simulink model "Galvo_sys_C__cont___Pcont_ccvc_FET_SUB_REF_v66"  (R2013a)
settings: Solver=ode23s  StartTime=0.0  StopTime=15e-3  FixedStep=FS  RelTol=1e-3
PreLoadFcn:
  | vname=@(x) inputname(1);
  | paramCtrl=evalin('base','paramCtrl;');
  | I_LIM=str2num(paramCtrl.I_LIM);
  | Kbc=str2num(paramCtrl.Kbc);
  | FS=evalin('base','FS;');
InitFcn:
  | %%%%%%  set scope time range
  | T_STOP=str2num(get_param(gcs,'StopTime'));
  | if numel(T_STOP) > 1
  |    T_STOP=T_STOP(2);
  | else
  |    T_STOP=T_STOP(1);
  | end
  | T_STOP=num2str(T_STOP);
  | 
  | %%%%%%  set scope time range in system @init_callback_fct
  | T_STOP=num2str(str2num(get_param(gcs,'StopTime')));
  | 
  | childs = allchild(0);
  | sol=strfind(upper(get(allchild(0),'Tag')),'VIEWER_PARAMETERS');
  | 
  | if iscell(sol)
  |    ind=find(~cellfun(@isempty, strfind(upper(get(allchild(0),'Tag')),'VIEWER_PARAMETERS')));
  | else
  |    ind=sol;
  | end
  | %ind=find(~cellfun(@isempty, {strfind(upper(get(allchild(0),'Tag')),'VIEWER_PARAMETERS'),[]}))
  | if ~isempty(ind)
  |    for k=1:length(childs(ind))
  |       set_param(getfield(get(childs(ind(k)),'UserData'),'block'),'TimeRange',T_STOP);
  |       get_param(getfield(get(childs(ind(k)),'UserData'),'block'),'TimeRange');
  | %    set_param(getfield(get(childs(ind),'UserData'),'block'),'TimeRange',T_STOP);
  | %    get_param(getfield(get(childs(ind),'UserData'),'block'),'TimeRange');
  |    end
  | else
  |     warning(sprintf('VIEWER_PARAMETERS object not found\nOpen the config dialog by hand for the first sim start'))
  | end
  | 
  | 
  | ADCres = str2num(get_param(gcs,'ADCres'));
  | Aref = str2num(get_param(gcs,'Aref'));
StartFcn:
  | I_LIM=str2num(paramCtrl.I_LIM);
  | Kbc=str2num(paramCtrl.Kbc);
  | %FS=evalin('base','FS;');
  | 
  | 
  | ADCres = str2num(get_param(gcs,'ADCres'));
  | Aref = str2num(get_param(gcs,'Aref'));
undefined symbols (not defined in the file or in its folder): ccG0, JR, KBM, KFR, KMT, KTB, Lc, Rc, Rsh
libraries: simulink x10, dspsigops x1
Description:
  | Eigentlich sollte in diesem Modell als current comp. ein ref. block mit zwei Varianten "alte 12V endstufe" und "neue 30V endstufe" eingesetzt werden. Sobald ein subsystem als referenced model eingesetzt wird, kommen die warnungen wegen algebr. schleifen obwohl sich die Blockdiagramme nicht unterscheiden.
  | --> anstatt "referenced variants" kommt halt wieder ein "subsystem variants" block als
  | cc rein...
settings Model: Aref=2.5  ADCres=12  BufferReuse=off  Creator=mainster  LastModifiedBy=mainster
settings SolverCC: AutoInsertRateTranBlk=on
settings DataIOCC: LimitDataPoints=off  SaveOutput=off  SaveTime=off
settings OptimizationCC: BlockReduction=off  InlineParams=on  OptimizeBlockIOStorage=off  BufferReuse=off  ExpressionFolding=off  LocalBlockOutputs=off
settings DebuggingCC: SolverPrmCheckMsg=none  InitInArrayFormatMsg=none
settings ModelReferenceCC: ModelReferenceNumInstancesAllowed=Single  ModelReferenceMinAlgLoopOccurrences=on

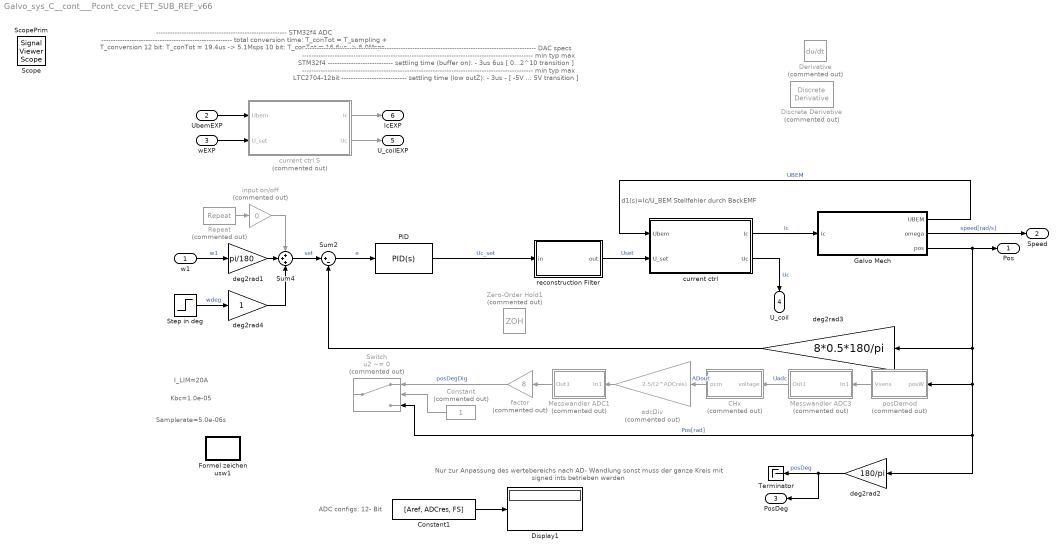
== system Galvo_sys_C__cont___Pcont_ccvc_FET_SUB_REF_v66 ==
  note: --------------------------------------------------------
      |  STM32f4 	ADC
      | --------------------------------------------------------
      | total conversion time:
      | T_conTot = T_sampling + T_conversion
      |
      | 12 bit: T_conTot = 19.4us -> 5.1Msps
      | 10 bit: T_conTot = 16.6us -> 6.0Msps
  note: Nur zur Anpassung des wertebereichs nach AD- Wandlung
      | sonst muss der ganze Kreis mit signed ints betrieben werden
  note: I_LIM=20A
  note: Kbc=1.0e-05
  note: Samplerate=5.0e-06s
  note: d1(s)=Ic/U_BEM
      | Stellfehler durch BackEMF
  note: ADC configs:
      | 12- Bit
  note: ---------------------------------------------------------------------------------------------------
      |  DAC specs
      | ---------------------------------------------------------------------------------------------------
      | 										min	typ		max
      | STM32f4							  ----------------------------
      | settling time (buffer on):	   -		3us	6us	[ 0...2^10 transition ]
      |
      | ---------------------------------------------------------------------------------------------------
      | 										min	typ		max
      | LTC2704-12bit 					  ----------------------------
      | settling time (low outZ):	   -		3us	-		[ -5V ... 5V transition ]
  w1 : Inport
  UbemEXP : Inport  Port=2
  wEXP : Inport  Port=3
  CHx : Subsystem  Commented=on  mask{bypass=off, N=eval(get_param(gcs,'ADCres'))}
      mask prompts: bypass "bypass adc"; N "Resolution"
      mask Callback bypass: %Simulink.Block.eval([gcb '/switch']);
      mask Callback N:
      | %va=strsplit(get_param(gcb, 'MaskVariables'), ';');
      | %ind=find(~cellfun(@isempty, strfind(va,'N')));
      | %sp=strsplit(va{ind},'=');
      | %@1
      | %set_param(gcs,'ADCres', @1)
      | %get_param(gcb, 'MaskVariables')
      mask Display:
      | %fprintf('ADC\nGain=%s\n=%i',...
      | %    get_param([gcb '/scale'], 'Gain'),...
      | %    eval( get_param([gcb '/scale'], 'Gain') ));
      | if bypass
      |     color('red')
      |     fprintf('bypass\nADC\n%i Bit', N)
      | else
      |     color('black')
      |     fprintf('ADC\n%i Bit', N)
      | end
  Constant : Constant  Commented=on
  Constant1 : Constant  Value=[Aref, ADCres, FS]
  Derivative : Derivative  Commented=on
  Discrete Derivative : simulink/Discrete/Discrete Derivative  Commented=on  gainval=1.0  ICPrevScaledInput=0.0  InputProcessing=Inherited  OutMin=[]  OutMax=[]  OutDataType=fixdt(1, 16)  OutScaling=2^-10  DoSatur=off
  Display1 : Display
  Formel zeichen usw1 : Subsystem
  Galvo Mech : Subsystem
  Messwandler ADC1 : Subsystem  Commented=on  mask{bias=-1.25, fact=1}
      mask prompts: bias "Enter offset"; fact "factor"
      mask TypeOptions bias: bias/Value
      mask TypeOptions fact: input div/Gain
      mask Display:
      | if bias < 0
      |     fprintf('y=%.4g*x%.4g',fact,bias)
      | else
      |     fprintf('y=%.4g*x+%.4g',fact,bias)
      | end
      | %port_label('input', 1, 'Vsens','texmode','off')
      | %port_label('output', 1, 'Vadc','texmode','off')
  Messwandler ADC3 : Subsystem  Commented=on  mask{bias=1.25, fact=1/4}
      mask prompts: bias "Enter offset"; fact "factor"
      mask TypeOptions bias: bias/Value
      mask TypeOptions fact: input div/Gain
      mask Display:
      | if bias < 0
      |     fprintf('y=%.4g*x%.4g',fact,bias)
      | else
      |     fprintf('y=%.4g*x+%.4g',fact,bias)
      | end
      | %port_label('input', 1, 'Vsens','texmode','off')
      | %port_label('output', 1, 'Vadc','texmode','off')
  PID : simulink/Continuous/PID Controller  OverrideUsingVariant=Ccc_no_vc  Controller=PID  TimeDomain=Continuous-time  SampleTime=FS  IntegratorMethod=Forward Euler  FilterMethod=Forward Euler  Form=Ideal  P=0.07188855202767  I=16.9554969036776  D=0.00441728282330501  N=3631.54350011101  InitialConditionSource=internal  InitialConditionForIntegrator=0  InitialConditionForFilter=0  ExternalReset=none  IgnoreLimit=on  LimitOutput=on  UpperSaturationLimit=30  LowerSaturationLimit=-30  LinearizeAsGain=off  AntiWindupMode=clamping  Kb=0.1  TrackingMode=off  Kt=0  PParamMin=[]  PParamMax=[]  IParamMin=[]  IParamMax=[]  DParamMin=[]  DParamMax=[]  NParamMin=[]  NParamMax=[]  KbParamMin=[]  KbParamMax=[]  KtParamMin=[]  KtParamMax=[]  POutMin=[]  POutMax=[]  IOutMin=[]  IOutMax=[]  DOutMin=[]  DOutMax=[]  NOutMin=[]  NOutMax=[]  KbOutMin=[]  KbOutMax=[]  KtOutMin=[]  KtOutMax=[]  IntegratorOutMin=[]  IntegratorOutMax=[]  FilterOutMin=[]  FilterOutMax=[]  SumOutMin=[]  SumOutMax=[]  SumI1OutMin=[]  SumI1OutMax=[]  SumI2OutMin=[]  SumI2OutMax=[]  SumI3OutMin=[]  SumI3OutMax=[]  SumDOutMin=[]  SumDOutMax=[]  SaturationOutMin=[]  SaturationOutMax=[]  IntegratorContinuousStateAttributes=''  IntegratorStateMustResolveToSignalObject=off  IntegratorRTWStateStorageClass=Auto  FilterContinuousStateAttributes=''  FilterStateMustResolveToSignalObject=off  FilterRTWStateStorageClass=Auto
      settings: AttributesFormatString=UpLim:%<UpperSaturationLimit>\nLoLim:%<LowerSaturationLimit>
  Repeat : dspsigops/Repeat  Commented=on  N=length(str2num(get_param([gcs '/Sequence Stair'], 'OutValues')))  InputProcessing=Columns as channels (frame based)  RateOptions=Allow multirate processing  ic=0  mode=Unused parameter value
  Step in deg : Step  Time=1e-3  After=5  SampleTime=0  ZeroCross=off
      settings: AttributesFormatString=Ampl.: %<After>\ntime:%<Time>
  Sum2 : Sum  Inputs=|+-
  Sum4 : Sum  Inputs=+++
  Switch : Switch  Commented=on  Criteria=u2 ~= 0
  Terminator : Terminator
  Zero-Order Hold1 : ZeroOrderHold  Commented=on  SampleTime=FS
  adcDiv : Gain  Commented=on  Gain=2.5/(2^ADCres)
  current ctrl : Subsystem  Variant=on  OverrideUsingVariant=Ccc_blocks_est
  current ctrl S : Subsystem  Commented=on  Variant=on  OverrideUsingVariant=Ccc_blocks_est
  deg2rad1 : Gain  Gain=pi/180
  deg2rad2 : Gain  Gain=180/pi
  deg2rad3 : Gain  Gain=8*0.5*180/pi
  deg2rad4 : Gain
  factor : Gain  Commented=on  Gain=8
  input on/off : Gain  Commented=on  Gain=0  SampleTime=FS
  posDemod : Subsystem  Commented=on
      mask Display: fprintf('Angular\npos sens\n 0.5V/°')
  "reconstruction Filter " : Subsystem  Variant=on  OverrideUsingVariant=v1  mask{bypass=on}
      mask prompts: bypass "bypass reconstruction filter"
      mask Display:
      | %fprintf('ADC\nGain=%s\n=%i',...
      | %    get_param([gcb '/scale'], 'Gain'),...
      | %    eval( get_param([gcb '/scale'], 'Gain') ));
      | if bypass
      |     color('red')
      |     fprintf('bypass\nReconstr.\nFilter')
      | else
      |     color('black')
      |     fprintf('Reconstr.\nFilter')
      | end
  Pos : Outport
  Speed : Outport  Port=2
  PosDeg : Outport  Port=3
  U_coil : Outport  Port=4
  U_coilEXP : Outport  Port=5
  IcEXP : Outport  Port=6
  Scope : SignalViewerScope  IOType=viewer  NumInputPorts=5  ZoomMode=xonly  LegendLocations=|  RefreshTime=0.035000
      | 0.85023     0.92601     0.11223    0.044868
      | 0.85952     0.73835     0.10294    0.025189
      | 0.66447     0.53227     0.29799    0.044868
      | 0.83166     0.36429      0.1308    0.025189
      |       0           0           0           0
      settings: ShowLegends=on  TimeRange=0.015  YMin=-0.05~-0.05~0~-2.5~-5  YMax=0.45~0.45~0.15~22.5~5
  ScopePrim : SignalViewerScope  IOType=viewer  NumInputPorts=5  ZoomMode=xonly  LegendLocations=|  RefreshTime=0.033391
      | 0.73662     0.90556     0.18911    0.037382
      | 0.76983     0.74948     0.16697    0.020986
      | 0.81411     0.55955     0.12269    0.020986
      |  0.7809     0.35428     0.14483    0.020986
      | 0.76983     0.16435     0.11162    0.020986
      settings: ShowLegends=on  TimeRange=0.015  YMin=-2~-2~-4~-2~-100  YMax=6~6~8~6~400
  wires:
  w1/1 -> deg2rad1/1  "w1"
  Repeat/1 -> input on/off/1
  Sum2/1 -> PID/1  "e"
  Sum4/1 -> Sum2/1  "set"
  Step in deg/1 -> deg2rad4/1  "wdeg"
  input on/off/1 -> Sum4/1
  deg2rad2/1 -> PosDeg/1, Terminator/1  "posDeg"
  deg2rad1/1 -> Sum4/2
  PID/1 -> "reconstruction Filter "/1(in)  "Uc_set"
  current ctrl/2(Uc) -> U_coil/1  "Uc"
  Galvo Mech/3(pos) -> posDemod/1(posW), Switch/3, deg2rad2/1, deg2rad3/1, Pos/1  "Pos[rad]"
  current ctrl/1(Ic) -> Galvo Mech/1(Ic)  "Ic"
  Galvo Mech/2(omega) -> Speed/1  "speed[rad/s]"
  Galvo Mech/1(UBEM) -> current ctrl/1(Ubem)  "UBEM"
  posDemod/1(Vsens) -> Messwandler ADC3/1(In1)
  Messwandler ADC3/1(Out1) -> CHx/1(voltage)  "Uadc"
  CHx/1(pcm) -> adcDiv/1  "ADout"
  Messwandler ADC1/1(Out1) -> factor/1
  adcDiv/1 -> Messwandler ADC1/1(In1)
  Constant1/1 -> Display1/1
  factor/1 -> Switch/1  "posDegDig"
  "reconstruction Filter "/1(out) -> current ctrl/2(U_set)  "Uset"
  Constant/1 -> Switch/2
  UbemEXP/1 -> current ctrl S/1(Ubem)
  wEXP/1 -> current ctrl S/2(U_set)
  current ctrl S/1(Ic) -> IcEXP/1
  current ctrl S/2(Uc) -> U_coilEXP/1
  deg2rad4/1 -> Sum4/3
  deg2rad3/1 -> Sum2/2

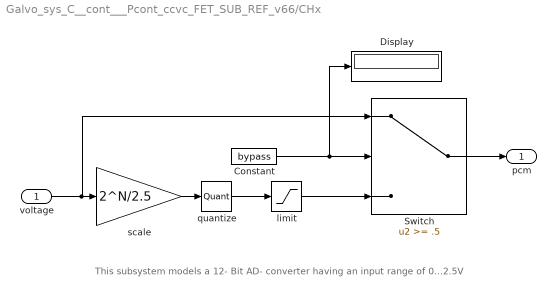
== system Galvo_sys_C__cont___Pcont_ccvc_FET_SUB_REF_v66/CHx ==
  note: This subsystem models a 12- Bit AD- converter
      | having an input  range of 0...2.5V
  voltage : Inport
  Constant : Constant  Value=bypass
  Display : Display
  Switch : Switch  Threshold=.5
  limit : Saturate  UpperLimit=2^N-1  LowerLimit=0
  quantize : Quantizer
  scale : Gain  Gain=2^N/2.5  SaturateOnIntegerOverflow=on  OutDataTypeStr=Inherit: Same as input  ParamDataTypeStr=Inherit: Same as input
  pcm : Outport
  wires:
  limit/1 -> Switch/3
  scale/1 -> quantize/1
  quantize/1 -> limit/1
  voltage/1 -> Switch/1, scale/1
  Constant/1 -> Display/1, Switch/2
  Switch/1 -> pcm/1

== system Galvo_sys_C__cont___Pcont_ccvc_FET_SUB_REF_v66/Formel zeichen usw1 ==
  note: Te: 		electrical torque, gen. by coils		[Nm]
      |  Ic: 			coil current							[A]
      |  Tfr:		rotor dynamic friction torque 		[Nm]
      |  Trb:		torsion bar torque					[Nm]
      |  Tw:		angular momentum				[Nm*s]
      |  w:			angular velocity 					[rad/s]
      |  yrad:		angular position 					[rad]
      |  ydeg:		angular position 					[°]
      |  Ucci:		current controller input				[V]
      |  Ucco:		current controller output			[V]
      |  Ush:		shunt voltage						[V]
  note: L_{c  }	coil inductance 							[H]
      |  R_{c  }	coil resistance							[\Omega]
      |  R_{SH }	current shunt resistance				[\Omega]
      |  J_{R  }	rotor inertia 							[kg*m²]
      |  K_{TB }	torsion bar torque const. 			[Nm/rad]
      |  K_{BM }	back EMF const.							[V*s/rad]
      |  K_{FR }	rotor dyn. friction torque const.	[Nm*s/rad]
      |  K_{MT }	el. magnetic torque const.			[Nm/A]
  note: balance of force: 	Te=Ttb+Tfr
      | 					Te - (Ttb+Tfr)=0  ->  no movement
      |
      |  integrate( 1 Nm )dt = 1 Nm*s
      |  (Nm*s)(kg*m²)⁻¹ = (N*s/kg)*m⁻¹ = m/(s*m) = rad

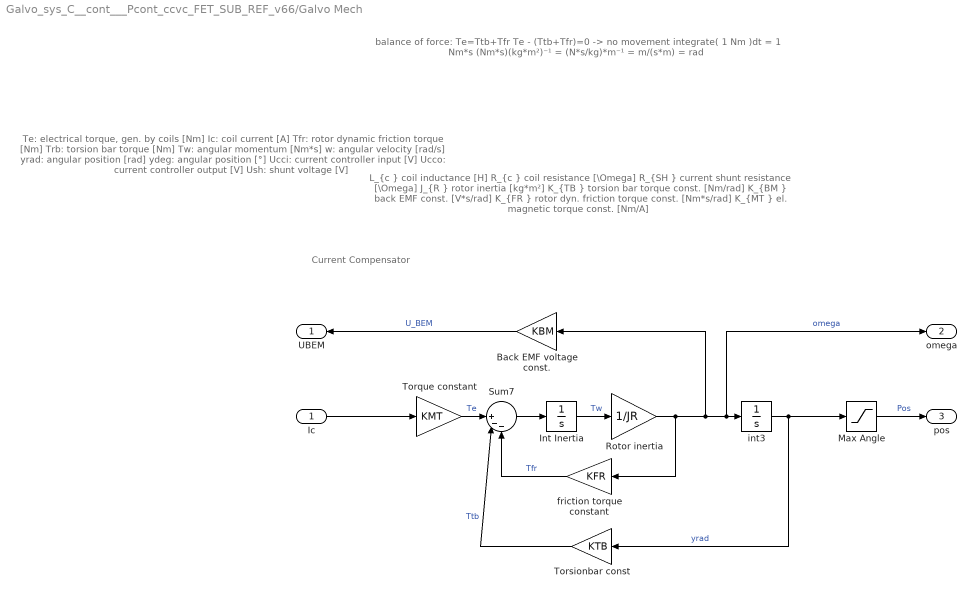
== system Galvo_sys_C__cont___Pcont_ccvc_FET_SUB_REF_v66/Galvo Mech ==
  note: Current Compensator
  note: Te: 		electrical torque, gen. by coils		[Nm]
      |  Ic: 			coil current							[A]
      |  Tfr:		rotor dynamic friction torque 		[Nm]
      |  Trb:		torsion bar torque					[Nm]
      |  Tw:		angular momentum				[Nm*s]
      |  w:			angular velocity 					[rad/s]
      |  yrad:		angular position 					[rad]
      |  ydeg:		angular position 					[°]
      |  Ucci:		current controller input				[V]
      |  Ucco:		current controller output			[V]
      |  Ush:		shunt voltage						[V]
  note: L_{c  }	coil inductance 							[H]
      |  R_{c  }	coil resistance							[\Omega]
      |  R_{SH }	current shunt resistance				[\Omega]
      |  J_{R  }	rotor inertia 							[kg*m²]
      |  K_{TB }	torsion bar torque const. 			[Nm/rad]
      |  K_{BM }	back EMF const.							[V*s/rad]
      |  K_{FR }	rotor dyn. friction torque const.	[Nm*s/rad]
      |  K_{MT }	el. magnetic torque const.			[Nm/A]
  note: balance of force: 	Te=Ttb+Tfr
      | 					Te - (Ttb+Tfr)=0  ->  no movement
      |
      |  integrate( 1 Nm )dt = 1 Nm*s
      |  (Nm*s)(kg*m²)⁻¹ = (N*s/kg)*m⁻¹ = m/(s*m) = rad
  Ic : Inport
  Back EMF voltage const. : Gain  Gain=KBM
  Int Inertia : Integrator
  Max Angle : Saturate  UpperLimit=20  LowerLimit=-20
      settings: AttributesFormatString=Max=%<UpperLimit>\nMin=%<LowerLimit>
  Rotor inertia : Gain  Gain=1/JR
  Sum7 : Sum  Inputs=||+--
  Torque constant : Gain  Gain=KMT
  Torsionbar const : Gain  Gain=KTB
  friction torque constant : Gain  Gain=KFR
  int3 : Integrator
  UBEM : Outport
  omega : Outport  Port=2
  pos : Outport  Port=3
  wires:
  Int Inertia/1 -> Rotor inertia/1  "Tw"
  Max Angle/1 -> pos/1  "Pos"
  Torsionbar const/1 -> Sum7/2  "Ttb"
  Sum7/1 -> Int Inertia/1
  Back EMF voltage const./1 -> UBEM/1  "U_BEM"
  int3/1 -> Max Angle/1, Torsionbar const/1  "yrad"
  Rotor inertia/1 -> omega/1, int3/1, Back EMF voltage const./1, friction torque constant/1  "omega"
  Torque constant/1 -> Sum7/1  "Te"
  friction torque constant/1 -> Sum7/3  "Tfr"
  Ic/1 -> Torque constant/1

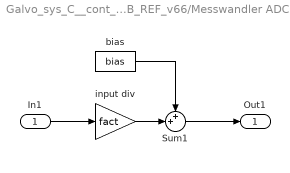
== system Galvo_sys_C__cont___Pcont_ccvc_FET_SUB_REF_v66/Messwandler ADC1 ==
  In1 : Inport
  Sum1 : Sum  Inputs=++|
  bias : Constant  Value=bias
  input div : Gain  Gain=fact
  Out1 : Outport
  wires:
  In1/1 -> input div/1
  bias/1 -> Sum1/1
  Sum1/1 -> Out1/1
  input div/1 -> Sum1/2

== system Galvo_sys_C__cont___Pcont_ccvc_FET_SUB_REF_v66/Messwandler ADC3 ==
  In1 : Inport
  Sum1 : Sum  Inputs=++|
  bias : Constant  Value=bias
  input div : Gain  Gain=fact
  Out1 : Outport
  wires:
  In1/1 -> input div/1
  bias/1 -> Sum1/1
  Sum1/1 -> Out1/1
  input div/1 -> Sum1/2

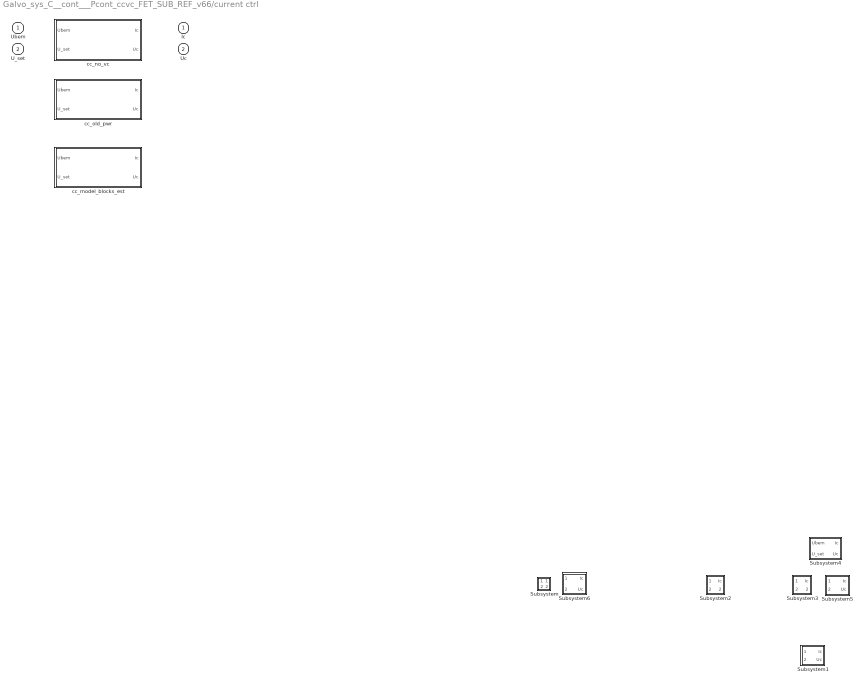
== system Galvo_sys_C__cont___Pcont_ccvc_FET_SUB_REF_v66/current ctrl ==
  Ubem : Inport
  U_set : Inport  Port=2
  Subsystem : Subsystem  VariantControl=Variant
  Subsystem1 : Subsystem  VariantControl=Variant2
  Subsystem2 : Subsystem  VariantControl=Variant3
  Subsystem3 : Subsystem  VariantControl=Variant4
  Subsystem4 : Subsystem  VariantControl=Variant5
  Subsystem5 : Subsystem  VariantControl=Variant6
  Subsystem6 : Subsystem  VariantControl=Variant7
  cc_model_blocks_est : Subsystem  VariantControl=Ccc_blocks_est
  cc_no_vc : Subsystem  VariantControl=Ccc_no_vc
  cc_old_pwr : Subsystem  VariantControl=Ccc_old_pwr
  Ic : Outport
  Uc : Outport  Port=2

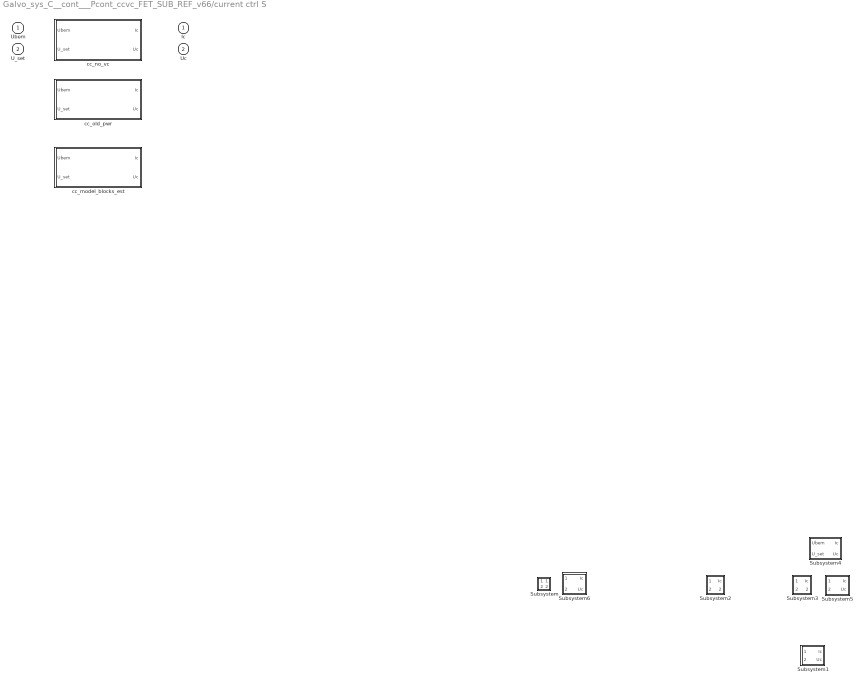
== system Galvo_sys_C__cont___Pcont_ccvc_FET_SUB_REF_v66/current ctrl S ==
  Ubem : Inport
  U_set : Inport  Port=2
  Subsystem : Subsystem  VariantControl=Variant
  Subsystem1 : Subsystem  VariantControl=Variant2
  Subsystem2 : Subsystem  VariantControl=Variant3
  Subsystem3 : Subsystem  VariantControl=Variant4
  Subsystem4 : Subsystem  VariantControl=Variant5
  Subsystem5 : Subsystem  VariantControl=Variant6
  Subsystem6 : Subsystem  VariantControl=Variant7
  cc_model_blocks_est : Subsystem  VariantControl=Ccc_blocks_est
  cc_no_vc : Subsystem  VariantControl=Ccc_no_vc
  cc_old_pwr : Subsystem  VariantControl=Ccc_old_pwr
  Ic : Outport
  Uc : Outport  Port=2

== system Galvo_sys_C__cont___Pcont_ccvc_FET_SUB_REF_v66/posDemod ==
  note: PosDemod übersetzt pos=+-20° in Vsens=+-10V
      | Skalierung: 0.5V/deg
      |
      | Der rad2deg block wird benötigt, weil sich die System-
      | dgls auf die Kreisfrequenz beziehen !!!
      | Ab hier ist die Einheit des Signal der Winkelposition deg
      | \color{red}und das bleibt auch so --> \bf Sollwert in deg
  posW : Inport
  rad2deg : Gain  Gain=180/pi
  scale : Gain  Gain=0.5
  Vsens : Outport
  wires:
  posW/1 -> rad2deg/1
  scale/1 -> Vsens/1
  rad2deg/1 -> scale/1

== system Galvo_sys_C__cont___Pcont_ccvc_FET_SUB_REF_v66/reconstruction Filter  ==
  in : Inport
  "reconstruct. Filter - DAC " : Subsystem  VariantControl=v1
  reconstruct. Filter - DAC 1 : Subsystem  VariantControl=bypass
  out : Outport

== system Galvo_sys_C__cont___Pcont_ccvc_FET_SUB_REF_v66/current ctrl/Subsystem ==
  Ubem : Inport
  U_set : Inport  Port=2
  Sum1 : Sum  Inputs=|+-
  Ic : Outport
  Uc : Outport  Port=2

== system Galvo_sys_C__cont___Pcont_ccvc_FET_SUB_REF_v66/current ctrl/Subsystem1 ==
  Ubem : Inport
  U_set : Inport  Port=2
  Shunt res.1 : Gain  Gain=Rsh
  Ic : Outport
  Uc : Outport  Port=2

== system Galvo_sys_C__cont___Pcont_ccvc_FET_SUB_REF_v66/current ctrl/Subsystem2 ==
  Ubem : Inport
  U_set : Inport  Port=2
  Plant SAT1 : Saturate  UpperLimit=15  LowerLimit=-15
      settings: AttributesFormatString=U_lim=+-%<UpperLimit>V
  Ic : Outport
  Uc : Outport  Port=2

== system Galvo_sys_C__cont___Pcont_ccvc_FET_SUB_REF_v66/current ctrl/Subsystem3 ==
  Ubem : Inport
  U_set : Inport  Port=2
  Int Coil : Integrator
  Ic : Outport
  Uc : Outport  Port=2

== system Galvo_sys_C__cont___Pcont_ccvc_FET_SUB_REF_v66/current ctrl/Subsystem4 ==
  Ubem : Inport
  U_set : Inport  Port=2
  Coil/Shunt res. : Gain  Gain=Rc+Rsh
  Ic : Outport
  Uc : Outport  Port=2

== system Galvo_sys_C__cont___Pcont_ccvc_FET_SUB_REF_v66/current ctrl/Subsystem5 ==
  Ubem : Inport
  U_set : Inport  Port=2
  Coil Inductance : Gain  Gain=1/Lc
  Ic : Outport
  Uc : Outport  Port=2

== system Galvo_sys_C__cont___Pcont_ccvc_FET_SUB_REF_v66/current ctrl/Subsystem6 ==
  Ubem : Inport
  U_set : Inport  Port=2
  Cc(s) : simulink/Continuous/PID Controller  Controller=P  TimeDomain=Continuous-time  SampleTime=-1  IntegratorMethod=Forward Euler  FilterMethod=Forward Euler  Form=Ideal  P=3.52446212597481  I=14078.2261040339  D=0  N=100  InitialConditionSource=internal  InitialConditionForIntegrator=0  InitialConditionForFilter=0  ExternalReset=none  LimitOutput=off  UpperSaturationLimit=inf  LowerSaturationLimit=-inf  LinearizeAsGain=on  AntiWindupMode=none  Kb=1  TrackingMode=off  Kt=1  PParamMin=[]  PParamMax=[]  IParamMin=[]  IParamMax=[]  DParamMin=[]  DParamMax=[]  NParamMin=[]  NParamMax=[]  KbParamMin=[]  KbParamMax=[]  KtParamMin=[]  KtParamMax=[]  POutMin=[]  POutMax=[]  IOutMin=[]  IOutMax=[]  DOutMin=[]  DOutMax=[]  NOutMin=[]  NOutMax=[]  KbOutMin=[]  KbOutMax=[]  KtOutMin=[]  KtOutMax=[]  IntegratorOutMin=[]  IntegratorOutMax=[]  FilterOutMin=[]  FilterOutMax=[]  SumOutMin=[]  SumOutMax=[]  SumI1OutMin=[]  SumI1OutMax=[]  SumI2OutMin=[]  SumI2OutMax=[]  SumI3OutMin=[]  SumI3OutMax=[]  SumDOutMin=[]  SumDOutMax=[]  SaturationOutMin=[]  SaturationOutMax=[]  IntegratorContinuousStateAttributes=''  IntegratorStateMustResolveToSignalObject=off  IntegratorRTWStateStorageClass=Auto  FilterContinuousStateAttributes=''  FilterStateMustResolveToSignalObject=off  FilterRTWStateStorageClass=Auto
  Ic : Outport
  Uc : Outport  Port=2

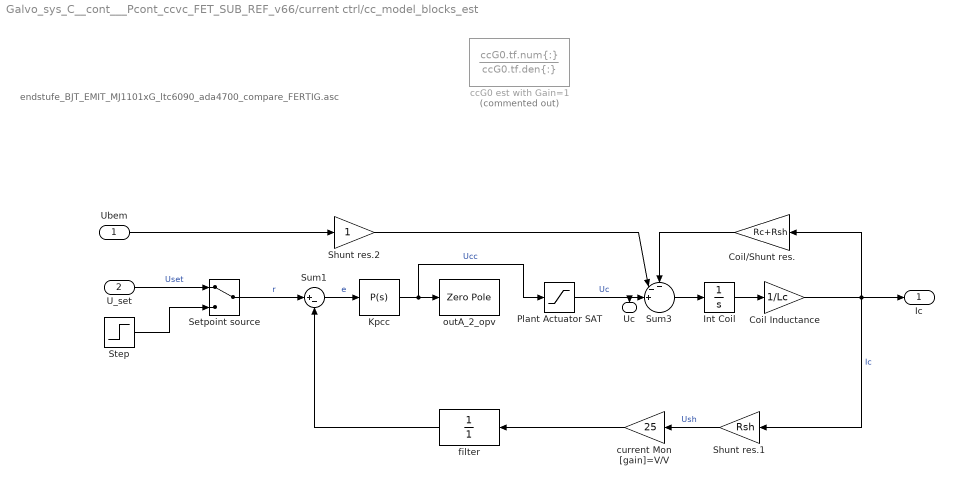
== system Galvo_sys_C__cont___Pcont_ccvc_FET_SUB_REF_v66/current ctrl/cc_model_blocks_est ==
  note: endstufe_BJT_EMIT_MJ1101xG_ltc6090_ada4700_compare_FERTIG.asc
  Ubem : Inport
  U_set : Inport  Port=2
  Coil Inductance : Gain  Gain=1/Lc
  Coil/Shunt res. : Gain  Gain=Rc+Rsh
  Int Coil : Integrator
  Kpcc : simulink/Continuous/PID Controller  Controller=P  TimeDomain=Continuous-time  SampleTime=-1  IntegratorMethod=Forward Euler  FilterMethod=Forward Euler  Form=Ideal  P=50  I=14078.2261040339  D=0  N=100  InitialConditionSource=internal  InitialConditionForIntegrator=0  InitialConditionForFilter=0  ExternalReset=none  LimitOutput=on  UpperSaturationLimit=30  LowerSaturationLimit=-30  LinearizeAsGain=on  AntiWindupMode=none  Kb=1  TrackingMode=off  Kt=1  PParamMin=[]  PParamMax=[]  IParamMin=[]  IParamMax=[]  DParamMin=[]  DParamMax=[]  NParamMin=[]  NParamMax=[]  KbParamMin=[]  KbParamMax=[]  KtParamMin=[]  KtParamMax=[]  POutMin=[]  POutMax=[]  IOutMin=[]  IOutMax=[]  DOutMin=[]  DOutMax=[]  NOutMin=[]  NOutMax=[]  KbOutMin=[]  KbOutMax=[]  KtOutMin=[]  KtOutMax=[]  IntegratorOutMin=[]  IntegratorOutMax=[]  FilterOutMin=[]  FilterOutMax=[]  SumOutMin=[]  SumOutMax=[]  SumI1OutMin=[]  SumI1OutMax=[]  SumI2OutMin=[]  SumI2OutMax=[]  SumI3OutMin=[]  SumI3OutMax=[]  SumDOutMin=[]  SumDOutMax=[]  SaturationOutMin=[]  SaturationOutMax=[]  IntegratorContinuousStateAttributes=''  IntegratorStateMustResolveToSignalObject=off  IntegratorRTWStateStorageClass=Auto  FilterContinuousStateAttributes=''  FilterStateMustResolveToSignalObject=off  FilterRTWStateStorageClass=Auto
      settings: AttributesFormatString=Kp=%<P>
  Plant Actuator SAT : Saturate  UpperLimit=30  LowerLimit=-30
      settings: AttributesFormatString=U_lim=+-%<UpperLimit>V
  Setpoint source : ManualSwitch
  Shunt res.1 : Gain  Gain=Rsh
  Shunt res.2 : Gain
  Step : Step  Time=1e-3  SampleTime=0
  Sum1 : Sum  Inputs=|+-
  Sum3 : Sum  Inputs=--+||
  ccG0 est with Gain=1 : TransferFcn  Commented=on  Numerator=ccG0.tf.num{:}  Denominator=ccG0.tf.den{:}
      settings: AttributesFormatString=%<numerator>\n%<denominator>
  current Mon [gain]=V/V : Gain  Gain=25
  filter : TransferFcn  Denominator=1
  outA_2_opv : ZeroPole  Zeros=3.4653e+08  Poles=-2.6678e+08  Gain=-0.7684
  Ic : Outport
  Uc : Outport  Port=2
  wires:
  Sum1/1 -> Kpcc/1  "e"
  Coil Inductance/1 -> Ic/1, Shunt res.1/1, Coil/Shunt res./1  "Ic"
  Plant Actuator SAT/1 -> Uc/1, Sum3/3  "Uc"
  Coil/Shunt res./1 -> Sum3/1
  Sum3/1 -> Int Coil/1
  Int Coil/1 -> Coil Inductance/1
  Shunt res.1/1 -> current Mon [gain]=V/V/1  "Ush"
  current Mon [gain]=V/V/1 -> filter/1
  Ubem/1 -> Shunt res.2/1
  U_set/1 -> Setpoint source/1  "Uset"
  Step/1 -> Setpoint source/2
  Setpoint source/1 -> Sum1/1  "r"
  Kpcc/1 -> Plant Actuator SAT/1, outA_2_opv/1  "Ucc"
  filter/1 -> Sum1/2
  Shunt res.2/1 -> Sum3/2

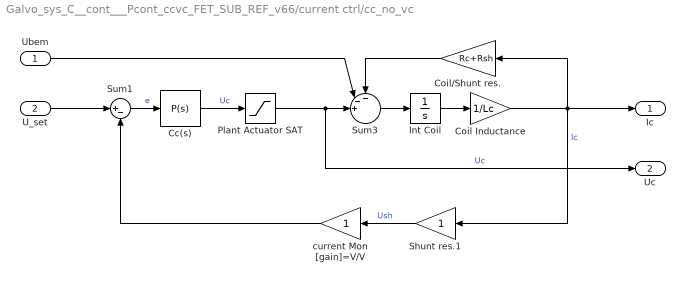
== system Galvo_sys_C__cont___Pcont_ccvc_FET_SUB_REF_v66/current ctrl/cc_no_vc ==
  Ubem : Inport
  U_set : Inport  Port=2
  Cc(s) : simulink/Continuous/PID Controller  Controller=P  TimeDomain=Continuous-time  SampleTime=-1  IntegratorMethod=Forward Euler  FilterMethod=Forward Euler  Form=Ideal  P=6.3432542926282  I=14078.2261040339  D=0  N=100  InitialConditionSource=internal  InitialConditionForIntegrator=0  InitialConditionForFilter=0  ExternalReset=none  LimitOutput=off  UpperSaturationLimit=inf  LowerSaturationLimit=-inf  LinearizeAsGain=on  AntiWindupMode=none  Kb=1  TrackingMode=off  Kt=1  PParamMin=[]  PParamMax=[]  IParamMin=[]  IParamMax=[]  DParamMin=[]  DParamMax=[]  NParamMin=[]  NParamMax=[]  KbParamMin=[]  KbParamMax=[]  KtParamMin=[]  KtParamMax=[]  POutMin=[]  POutMax=[]  IOutMin=[]  IOutMax=[]  DOutMin=[]  DOutMax=[]  NOutMin=[]  NOutMax=[]  KbOutMin=[]  KbOutMax=[]  KtOutMin=[]  KtOutMax=[]  IntegratorOutMin=[]  IntegratorOutMax=[]  FilterOutMin=[]  FilterOutMax=[]  SumOutMin=[]  SumOutMax=[]  SumI1OutMin=[]  SumI1OutMax=[]  SumI2OutMin=[]  SumI2OutMax=[]  SumI3OutMin=[]  SumI3OutMax=[]  SumDOutMin=[]  SumDOutMax=[]  SaturationOutMin=[]  SaturationOutMax=[]  IntegratorContinuousStateAttributes=''  IntegratorStateMustResolveToSignalObject=off  IntegratorRTWStateStorageClass=Auto  FilterContinuousStateAttributes=''  FilterStateMustResolveToSignalObject=off  FilterRTWStateStorageClass=Auto
  Coil Inductance : Gain  Gain=1/Lc
  Coil/Shunt res. : Gain  Gain=Rc+Rsh
  Int Coil : Integrator
  Plant Actuator SAT : Saturate  UpperLimit=30  LowerLimit=-30
      settings: AttributesFormatString=U_lim=+-%<UpperLimit>A
  Shunt res.1 : Gain
  Sum1 : Sum  Inputs=|+-
  Sum3 : Sum  Inputs=--+||
  current Mon [gain]=V/V : Gain
  Ic : Outport
  Uc : Outport  Port=2
  wires:
  Sum3/1 -> Int Coil/1
  Cc(s)/1 -> Plant Actuator SAT/1  "Uc"
  Coil/Shunt res./1 -> Sum3/1
  Ubem/1 -> Sum3/2
  Int Coil/1 -> Coil Inductance/1
  Coil Inductance/1 -> Coil/Shunt res./1, Shunt res.1/1, Ic/1  "Ic"
  Shunt res.1/1 -> current Mon [gain]=V/V/1  "Ush"
  Plant Actuator SAT/1 -> Sum3/3, Uc/1  "Uc"
  U_set/1 -> Sum1/1
  current Mon [gain]=V/V/1 -> Sum1/2
  Sum1/1 -> Cc(s)/1  "e"

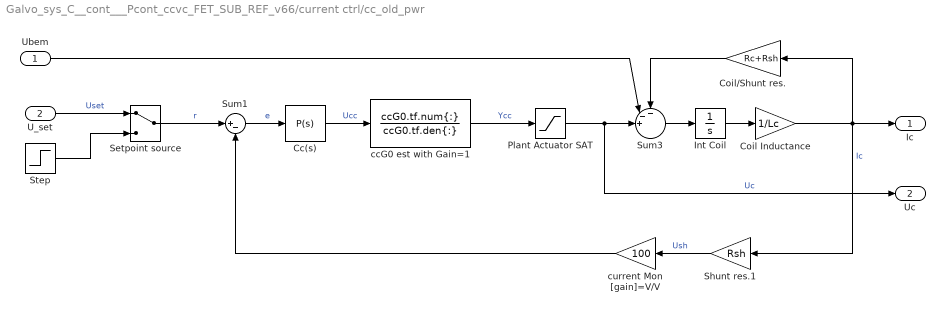
== system Galvo_sys_C__cont___Pcont_ccvc_FET_SUB_REF_v66/current ctrl/cc_old_pwr ==
  Ubem : Inport
  U_set : Inport  Port=2
  Cc(s) : simulink/Continuous/PID Controller  Controller=P  TimeDomain=Continuous-time  SampleTime=-1  IntegratorMethod=Forward Euler  FilterMethod=Forward Euler  Form=Ideal  P=3.52446212597481  I=14078.2261040339  D=0  N=100  InitialConditionSource=internal  InitialConditionForIntegrator=0  InitialConditionForFilter=0  ExternalReset=none  LimitOutput=off  UpperSaturationLimit=inf  LowerSaturationLimit=-inf  LinearizeAsGain=on  AntiWindupMode=none  Kb=1  TrackingMode=off  Kt=1  PParamMin=[]  PParamMax=[]  IParamMin=[]  IParamMax=[]  DParamMin=[]  DParamMax=[]  NParamMin=[]  NParamMax=[]  KbParamMin=[]  KbParamMax=[]  KtParamMin=[]  KtParamMax=[]  POutMin=[]  POutMax=[]  IOutMin=[]  IOutMax=[]  DOutMin=[]  DOutMax=[]  NOutMin=[]  NOutMax=[]  KbOutMin=[]  KbOutMax=[]  KtOutMin=[]  KtOutMax=[]  IntegratorOutMin=[]  IntegratorOutMax=[]  FilterOutMin=[]  FilterOutMax=[]  SumOutMin=[]  SumOutMax=[]  SumI1OutMin=[]  SumI1OutMax=[]  SumI2OutMin=[]  SumI2OutMax=[]  SumI3OutMin=[]  SumI3OutMax=[]  SumDOutMin=[]  SumDOutMax=[]  SaturationOutMin=[]  SaturationOutMax=[]  IntegratorContinuousStateAttributes=''  IntegratorStateMustResolveToSignalObject=off  IntegratorRTWStateStorageClass=Auto  FilterContinuousStateAttributes=''  FilterStateMustResolveToSignalObject=off  FilterRTWStateStorageClass=Auto
  Coil Inductance : Gain  Gain=1/Lc
  Coil/Shunt res. : Gain  Gain=Rc+Rsh
  Int Coil : Integrator
  Plant Actuator SAT : Saturate  UpperLimit=15  LowerLimit=-15
      settings: AttributesFormatString=U_lim=+-%<UpperLimit>V
  Setpoint source : ManualSwitch
  Shunt res.1 : Gain  Gain=Rsh
  Step : Step  SampleTime=0
  Sum1 : Sum  Inputs=|+-
  Sum3 : Sum  Inputs=--+||
  ccG0 est with Gain=1 : TransferFcn  Numerator=ccG0.tf.num{:}  Denominator=ccG0.tf.den{:}
      settings: AttributesFormatString=%<numerator>\n%<denominator>
  current Mon [gain]=V/V : Gain  Gain=100
  Ic : Outport
  Uc : Outport  Port=2
  wires:
  ccG0 est with Gain=1/1 -> Plant Actuator SAT/1  "Ycc"
  Sum1/1 -> Cc(s)/1  "e"
  Coil Inductance/1 -> Ic/1, Shunt res.1/1, Coil/Shunt res./1  "Ic"
  Plant Actuator SAT/1 -> Uc/1, Sum3/3  "Uc"
  Coil/Shunt res./1 -> Sum3/1
  Sum3/1 -> Int Coil/1
  Int Coil/1 -> Coil Inductance/1
  Cc(s)/1 -> ccG0 est with Gain=1/1  "Ucc"
  Shunt res.1/1 -> current Mon [gain]=V/V/1  "Ush"
  current Mon [gain]=V/V/1 -> Sum1/2
  Ubem/1 -> Sum3/2
  U_set/1 -> Setpoint source/1  "Uset"
  Step/1 -> Setpoint source/2
  Setpoint source/1 -> Sum1/1  "r"

== system Galvo_sys_C__cont___Pcont_ccvc_FET_SUB_REF_v66/current ctrl S/Subsystem ==
  Ubem : Inport
  U_set : Inport  Port=2
  Sum1 : Sum  Inputs=|+-
  Ic : Outport
  Uc : Outport  Port=2

== system Galvo_sys_C__cont___Pcont_ccvc_FET_SUB_REF_v66/current ctrl S/Subsystem1 ==
  Ubem : Inport
  U_set : Inport  Port=2
  Shunt res.1 : Gain  Gain=Rsh
  Ic : Outport
  Uc : Outport  Port=2

== system Galvo_sys_C__cont___Pcont_ccvc_FET_SUB_REF_v66/current ctrl S/Subsystem2 ==
  Ubem : Inport
  U_set : Inport  Port=2
  Plant SAT1 : Saturate  UpperLimit=15  LowerLimit=-15
      settings: AttributesFormatString=U_lim=+-%<UpperLimit>V
  Ic : Outport
  Uc : Outport  Port=2

== system Galvo_sys_C__cont___Pcont_ccvc_FET_SUB_REF_v66/current ctrl S/Subsystem3 ==
  Ubem : Inport
  U_set : Inport  Port=2
  Int Coil : Integrator
  Ic : Outport
  Uc : Outport  Port=2

== system Galvo_sys_C__cont___Pcont_ccvc_FET_SUB_REF_v66/current ctrl S/Subsystem4 ==
  Ubem : Inport
  U_set : Inport  Port=2
  Coil/Shunt res. : Gain  Gain=Rc+Rsh
  Ic : Outport
  Uc : Outport  Port=2

== system Galvo_sys_C__cont___Pcont_ccvc_FET_SUB_REF_v66/current ctrl S/Subsystem5 ==
  Ubem : Inport
  U_set : Inport  Port=2
  Coil Inductance : Gain  Gain=1/Lc
  Ic : Outport
  Uc : Outport  Port=2

== system Galvo_sys_C__cont___Pcont_ccvc_FET_SUB_REF_v66/current ctrl S/Subsystem6 ==
  Ubem : Inport
  U_set : Inport  Port=2
  Cc(s) : simulink/Continuous/PID Controller  Controller=P  TimeDomain=Continuous-time  SampleTime=-1  IntegratorMethod=Forward Euler  FilterMethod=Forward Euler  Form=Ideal  P=3.52446212597481  I=14078.2261040339  D=0  N=100  InitialConditionSource=internal  InitialConditionForIntegrator=0  InitialConditionForFilter=0  ExternalReset=none  LimitOutput=off  UpperSaturationLimit=inf  LowerSaturationLimit=-inf  LinearizeAsGain=on  AntiWindupMode=none  Kb=1  TrackingMode=off  Kt=1  PParamMin=[]  PParamMax=[]  IParamMin=[]  IParamMax=[]  DParamMin=[]  DParamMax=[]  NParamMin=[]  NParamMax=[]  KbParamMin=[]  KbParamMax=[]  KtParamMin=[]  KtParamMax=[]  POutMin=[]  POutMax=[]  IOutMin=[]  IOutMax=[]  DOutMin=[]  DOutMax=[]  NOutMin=[]  NOutMax=[]  KbOutMin=[]  KbOutMax=[]  KtOutMin=[]  KtOutMax=[]  IntegratorOutMin=[]  IntegratorOutMax=[]  FilterOutMin=[]  FilterOutMax=[]  SumOutMin=[]  SumOutMax=[]  SumI1OutMin=[]  SumI1OutMax=[]  SumI2OutMin=[]  SumI2OutMax=[]  SumI3OutMin=[]  SumI3OutMax=[]  SumDOutMin=[]  SumDOutMax=[]  SaturationOutMin=[]  SaturationOutMax=[]  IntegratorContinuousStateAttributes=''  IntegratorStateMustResolveToSignalObject=off  IntegratorRTWStateStorageClass=Auto  FilterContinuousStateAttributes=''  FilterStateMustResolveToSignalObject=off  FilterRTWStateStorageClass=Auto
  Ic : Outport
  Uc : Outport  Port=2

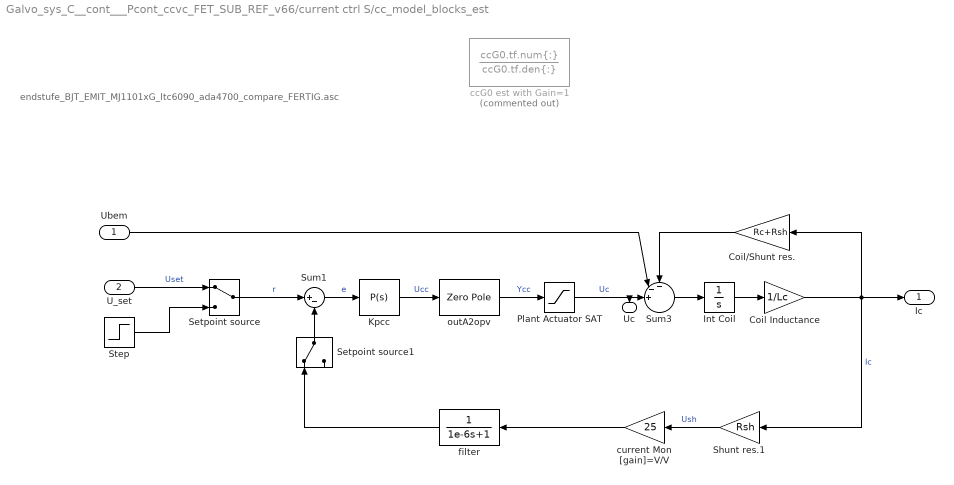
== system Galvo_sys_C__cont___Pcont_ccvc_FET_SUB_REF_v66/current ctrl S/cc_model_blocks_est ==
  note: endstufe_BJT_EMIT_MJ1101xG_ltc6090_ada4700_compare_FERTIG.asc
  Ubem : Inport
  U_set : Inport  Port=2
  Coil Inductance : Gain  Gain=1/Lc
  Coil/Shunt res. : Gain  Gain=Rc+Rsh
  Int Coil : Integrator
  Kpcc : simulink/Continuous/PID Controller  Controller=P  TimeDomain=Continuous-time  SampleTime=-1  IntegratorMethod=Forward Euler  FilterMethod=Forward Euler  Form=Ideal  P=200  I=14078.2261040339  D=0  N=100  InitialConditionSource=internal  InitialConditionForIntegrator=0  InitialConditionForFilter=0  ExternalReset=none  LimitOutput=off  UpperSaturationLimit=inf  LowerSaturationLimit=-inf  LinearizeAsGain=on  AntiWindupMode=none  Kb=1  TrackingMode=off  Kt=1  PParamMin=[]  PParamMax=[]  IParamMin=[]  IParamMax=[]  DParamMin=[]  DParamMax=[]  NParamMin=[]  NParamMax=[]  KbParamMin=[]  KbParamMax=[]  KtParamMin=[]  KtParamMax=[]  POutMin=[]  POutMax=[]  IOutMin=[]  IOutMax=[]  DOutMin=[]  DOutMax=[]  NOutMin=[]  NOutMax=[]  KbOutMin=[]  KbOutMax=[]  KtOutMin=[]  KtOutMax=[]  IntegratorOutMin=[]  IntegratorOutMax=[]  FilterOutMin=[]  FilterOutMax=[]  SumOutMin=[]  SumOutMax=[]  SumI1OutMin=[]  SumI1OutMax=[]  SumI2OutMin=[]  SumI2OutMax=[]  SumI3OutMin=[]  SumI3OutMax=[]  SumDOutMin=[]  SumDOutMax=[]  SaturationOutMin=[]  SaturationOutMax=[]  IntegratorContinuousStateAttributes=''  IntegratorStateMustResolveToSignalObject=off  IntegratorRTWStateStorageClass=Auto  FilterContinuousStateAttributes=''  FilterStateMustResolveToSignalObject=off  FilterRTWStateStorageClass=Auto
      settings: AttributesFormatString=Kp=%<P>
  Plant Actuator SAT : Saturate  UpperLimit=150  LowerLimit=-150
      settings: AttributesFormatString=U_lim=+-%<UpperLimit>V
  Setpoint source : ManualSwitch
  Setpoint source1 : ManualSwitch
  Shunt res.1 : Gain  Gain=Rsh
  Step : Step  SampleTime=0
  Sum1 : Sum  Inputs=|+-
  Sum3 : Sum  Inputs=--+||
  ccG0 est with Gain=1 : TransferFcn  Commented=on  Numerator=ccG0.tf.num{:}  Denominator=ccG0.tf.den{:}
      settings: AttributesFormatString=%<numerator>\n%<denominator>
  current Mon [gain]=V/V : Gain  Gain=25
  filter : TransferFcn  Denominator=[1e-6 1]
  outA2opv : ZeroPole  Zeros=3.4653e+08  Poles=-2.6678e+08  Gain=-0.7684
  Ic : Outport
  Uc : Outport  Port=2
  wires:
  outA2opv/1 -> Plant Actuator SAT/1  "Ycc"
  Sum1/1 -> Kpcc/1  "e"
  Coil Inductance/1 -> Ic/1, Shunt res.1/1, Coil/Shunt res./1  "Ic"
  Plant Actuator SAT/1 -> Uc/1, Sum3/3  "Uc"
  Coil/Shunt res./1 -> Sum3/1
  Sum3/1 -> Int Coil/1
  Int Coil/1 -> Coil Inductance/1
  Shunt res.1/1 -> current Mon [gain]=V/V/1  "Ush"
  current Mon [gain]=V/V/1 -> filter/1
  Ubem/1 -> Sum3/2
  U_set/1 -> Setpoint source/1  "Uset"
  Step/1 -> Setpoint source/2
  Setpoint source/1 -> Sum1/1  "r"
  Kpcc/1 -> outA2opv/1  "Ucc"
  filter/1 -> Setpoint source1/1
  Setpoint source1/1 -> Sum1/2

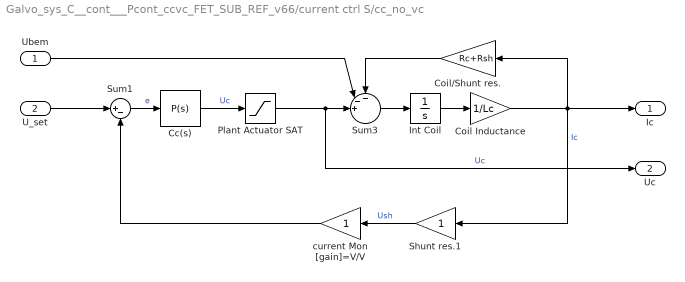
== system Galvo_sys_C__cont___Pcont_ccvc_FET_SUB_REF_v66/current ctrl S/cc_no_vc ==
  Ubem : Inport
  U_set : Inport  Port=2
  Cc(s) : simulink/Continuous/PID Controller  Controller=P  TimeDomain=Continuous-time  SampleTime=-1  IntegratorMethod=Forward Euler  FilterMethod=Forward Euler  Form=Ideal  P=6.3432542926282  I=14078.2261040339  D=0  N=100  InitialConditionSource=internal  InitialConditionForIntegrator=0  InitialConditionForFilter=0  ExternalReset=none  LimitOutput=off  UpperSaturationLimit=inf  LowerSaturationLimit=-inf  LinearizeAsGain=on  AntiWindupMode=none  Kb=1  TrackingMode=off  Kt=1  PParamMin=[]  PParamMax=[]  IParamMin=[]  IParamMax=[]  DParamMin=[]  DParamMax=[]  NParamMin=[]  NParamMax=[]  KbParamMin=[]  KbParamMax=[]  KtParamMin=[]  KtParamMax=[]  POutMin=[]  POutMax=[]  IOutMin=[]  IOutMax=[]  DOutMin=[]  DOutMax=[]  NOutMin=[]  NOutMax=[]  KbOutMin=[]  KbOutMax=[]  KtOutMin=[]  KtOutMax=[]  IntegratorOutMin=[]  IntegratorOutMax=[]  FilterOutMin=[]  FilterOutMax=[]  SumOutMin=[]  SumOutMax=[]  SumI1OutMin=[]  SumI1OutMax=[]  SumI2OutMin=[]  SumI2OutMax=[]  SumI3OutMin=[]  SumI3OutMax=[]  SumDOutMin=[]  SumDOutMax=[]  SaturationOutMin=[]  SaturationOutMax=[]  IntegratorContinuousStateAttributes=''  IntegratorStateMustResolveToSignalObject=off  IntegratorRTWStateStorageClass=Auto  FilterContinuousStateAttributes=''  FilterStateMustResolveToSignalObject=off  FilterRTWStateStorageClass=Auto
  Coil Inductance : Gain  Gain=1/Lc
  Coil/Shunt res. : Gain  Gain=Rc+Rsh
  Int Coil : Integrator
  Plant Actuator SAT : Saturate  UpperLimit=30  LowerLimit=-30
      settings: AttributesFormatString=U_lim=+-%<UpperLimit>A
  Shunt res.1 : Gain
  Sum1 : Sum  Inputs=|+-
  Sum3 : Sum  Inputs=--+||
  current Mon [gain]=V/V : Gain
  Ic : Outport
  Uc : Outport  Port=2
  wires:
  Sum3/1 -> Int Coil/1
  Cc(s)/1 -> Plant Actuator SAT/1  "Uc"
  Coil/Shunt res./1 -> Sum3/1
  Ubem/1 -> Sum3/2
  Int Coil/1 -> Coil Inductance/1
  Coil Inductance/1 -> Coil/Shunt res./1, Shunt res.1/1, Ic/1  "Ic"
  Shunt res.1/1 -> current Mon [gain]=V/V/1  "Ush"
  Plant Actuator SAT/1 -> Sum3/3, Uc/1  "Uc"
  U_set/1 -> Sum1/1
  current Mon [gain]=V/V/1 -> Sum1/2
  Sum1/1 -> Cc(s)/1  "e"

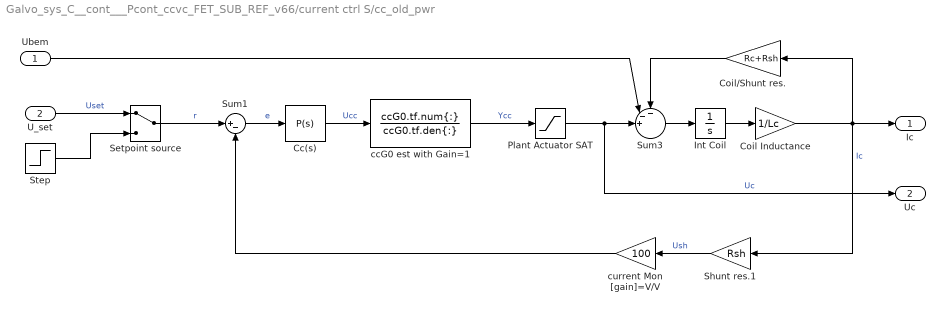
== system Galvo_sys_C__cont___Pcont_ccvc_FET_SUB_REF_v66/current ctrl S/cc_old_pwr ==
  Ubem : Inport
  U_set : Inport  Port=2
  Cc(s) : simulink/Continuous/PID Controller  Controller=P  TimeDomain=Continuous-time  SampleTime=-1  IntegratorMethod=Forward Euler  FilterMethod=Forward Euler  Form=Ideal  P=3.52446212597481  I=14078.2261040339  D=0  N=100  InitialConditionSource=internal  InitialConditionForIntegrator=0  InitialConditionForFilter=0  ExternalReset=none  LimitOutput=off  UpperSaturationLimit=inf  LowerSaturationLimit=-inf  LinearizeAsGain=on  AntiWindupMode=none  Kb=1  TrackingMode=off  Kt=1  PParamMin=[]  PParamMax=[]  IParamMin=[]  IParamMax=[]  DParamMin=[]  DParamMax=[]  NParamMin=[]  NParamMax=[]  KbParamMin=[]  KbParamMax=[]  KtParamMin=[]  KtParamMax=[]  POutMin=[]  POutMax=[]  IOutMin=[]  IOutMax=[]  DOutMin=[]  DOutMax=[]  NOutMin=[]  NOutMax=[]  KbOutMin=[]  KbOutMax=[]  KtOutMin=[]  KtOutMax=[]  IntegratorOutMin=[]  IntegratorOutMax=[]  FilterOutMin=[]  FilterOutMax=[]  SumOutMin=[]  SumOutMax=[]  SumI1OutMin=[]  SumI1OutMax=[]  SumI2OutMin=[]  SumI2OutMax=[]  SumI3OutMin=[]  SumI3OutMax=[]  SumDOutMin=[]  SumDOutMax=[]  SaturationOutMin=[]  SaturationOutMax=[]  IntegratorContinuousStateAttributes=''  IntegratorStateMustResolveToSignalObject=off  IntegratorRTWStateStorageClass=Auto  FilterContinuousStateAttributes=''  FilterStateMustResolveToSignalObject=off  FilterRTWStateStorageClass=Auto
  Coil Inductance : Gain  Gain=1/Lc
  Coil/Shunt res. : Gain  Gain=Rc+Rsh
  Int Coil : Integrator
  Plant Actuator SAT : Saturate  UpperLimit=15  LowerLimit=-15
      settings: AttributesFormatString=U_lim=+-%<UpperLimit>V
  Setpoint source : ManualSwitch
  Shunt res.1 : Gain  Gain=Rsh
  Step : Step  SampleTime=0
  Sum1 : Sum  Inputs=|+-
  Sum3 : Sum  Inputs=--+||
  ccG0 est with Gain=1 : TransferFcn  Numerator=ccG0.tf.num{:}  Denominator=ccG0.tf.den{:}
      settings: AttributesFormatString=%<numerator>\n%<denominator>
  current Mon [gain]=V/V : Gain  Gain=100
  Ic : Outport
  Uc : Outport  Port=2
  wires:
  ccG0 est with Gain=1/1 -> Plant Actuator SAT/1  "Ycc"
  Sum1/1 -> Cc(s)/1  "e"
  Coil Inductance/1 -> Ic/1, Shunt res.1/1, Coil/Shunt res./1  "Ic"
  Plant Actuator SAT/1 -> Uc/1, Sum3/3  "Uc"
  Coil/Shunt res./1 -> Sum3/1
  Sum3/1 -> Int Coil/1
  Int Coil/1 -> Coil Inductance/1
  Cc(s)/1 -> ccG0 est with Gain=1/1  "Ucc"
  Shunt res.1/1 -> current Mon [gain]=V/V/1  "Ush"
  current Mon [gain]=V/V/1 -> Sum1/2
  Ubem/1 -> Sum3/2
  U_set/1 -> Setpoint source/1  "Uset"
  Step/1 -> Setpoint source/2
  Setpoint source/1 -> Sum1/1  "r"

== system Galvo_sys_C__cont___Pcont_ccvc_FET_SUB_REF_v66/reconstruction Filter /reconstruct. Filter - DAC  ==
  note: Lp Sallenkey
      | Passband: 3kHz
      | Stopband: 10kHz = fs/2 @ Ts=50us
      | Stopband Dämpfung: -45dB
      | Delay: ~150us
  in : Inport
  Constant : Constant  Value=bypass
  Switch : Switch  Threshold=.5
  sallen key : TransferFcn  Numerator="[  0    0    0    0  5.36e+16  ]"  Denominator="[  1  2.31e+04  6.52e+08  7.55e+12  5.36e+16  ]"
  out : Outport
  wires:
  in/1 -> Switch/1, sallen key/1
  sallen key/1 -> Switch/3
  Constant/1 -> Switch/2
  Switch/1 -> out/1

== system Galvo_sys_C__cont___Pcont_ccvc_FET_SUB_REF_v66/reconstruction Filter /reconstruct. Filter - DAC 1 ==
  in : Inport
  out : Outport
  wires:
  in/1 -> out/1
